simulink model "thrust_model"  (R2018a)
settings: Solver=FixedStepAuto  StartTime=0.0  StopTime=t(end)  FixedStep=0.0104  RelTol=1e-3
settings Model: Creator=emran  LastModifiedBy=adiravishankara

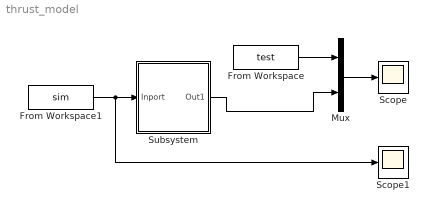
== system thrust_model ==
  From Workspace : FromWorkspace  VariableName=test  SampleTime=0.0104
  From Workspace1 : FromWorkspace  VariableName=sim  SampleTime=0.0104
  Mux : Mux  Inputs=2
  Scope : Scope
  Scope1 : Scope
  Subsystem : Subsystem
  wires:
  From Workspace1/1 -> Scope1/1, Subsystem/1(Inport)
  Subsystem/1(Out1) -> Mux/2
  From Workspace/1 -> Mux/1
  Mux/1 -> Scope/1

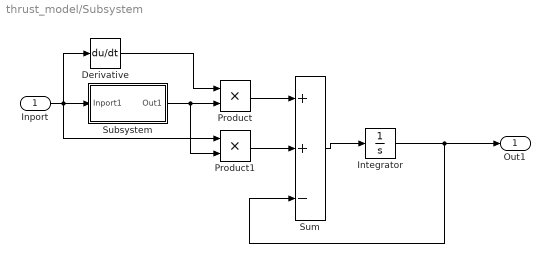
== system thrust_model/Subsystem ==
  Inport : Inport
  Derivative : Derivative
  Integrator : Integrator
  Product : Product
  Product1 : Product
  Subsystem : Subsystem
  Sum : Sum  Inputs=++-
  Out1 : Outport
  wires:
  Product/1 -> Sum/1
  Sum/1 -> Integrator/1
  Subsystem/1(Out1) -> Product1/2, Product/2
  Integrator/1 -> Sum/3, Out1/1
  Inport/1 -> Product1/1, Derivative/1, Subsystem/1(Inport1)
  Product1/1 -> Sum/2
  Derivative/1 -> Product/1

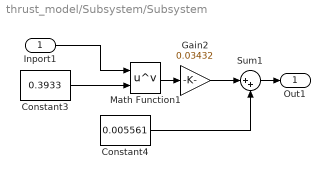
== system thrust_model/Subsystem/Subsystem ==
  Inport1 : Inport
  Constant3 : Constant  Value=0.3933
  Constant4 : Constant  Value=0.005561
  Gain2 : Gain  Gain=0.03432
  Math Function1 : Math  Operator=pow  SaturateOnIntegerOverflow=on
  Sum1 : Sum  Inputs=|++
  Out1 : Outport
  wires:
  Constant4/1 -> Sum1/2
  Sum1/1 -> Out1/1
  Math Function1/1 -> Gain2/1
  Inport1/1 -> Math Function1/1
  Gain2/1 -> Sum1/1
  Constant3/1 -> Math Function1/2
